simulink model "model_block"  (R2023a)
settings: Solver=VariableStepAuto  StartTime=0.0  StopTime=2  RelTol=1e-3
values from neighbouring files (symbols this model uses):
  C = 660e-6    (= 0.00066)    [execute_model.m]
  duty_cycle = 0.25    [execute_model.m]
  fsw = 15e3    (= 15000)    [execute_model.m]
  L = 200e-6    (= 0.0002)    [execute_model.m]
  R = 10    [execute_model.m]
  vin = 24    [execute_model.m]
libraries: simulink x1
settings Model: Creator=pablo  LastModifiedBy=pablo
settings OptimizationCC: ReuseModelBlockBuffer=off

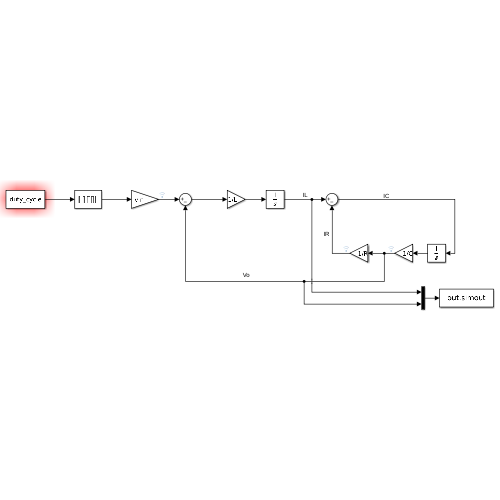
[thumbnail: Simulink's stored preview of the top-level diagram]
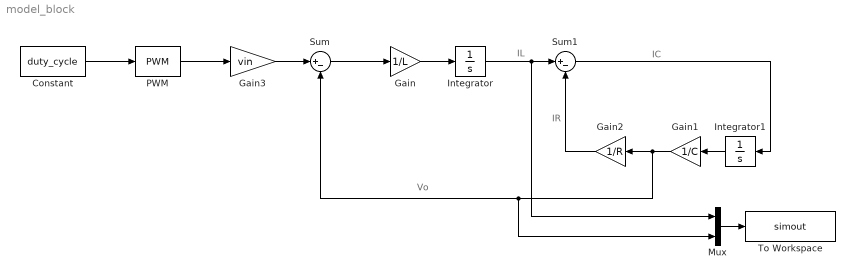
== system model_block ==
  note: IL
  note: IC
  note: IR
  note: Vo
  Constant : Constant  Value=duty_cycle
  Gain : Gain  Gain=1/L
  Gain1 : Gain  Gain=1/C
  Gain2 : Gain  Gain=1/R
  Gain3 : Gain  Gain=vin
  Integrator : Integrator
  Integrator1 : Integrator
  Mux : Mux  Inputs=2
  PWM : simulink/Discontinuities/PWM  DisableCoverage=on  Period=1/fsw  InitialDelay=0  DisallowZeroDutyCycle=off  RunAtFixedTimeIntervals=off  SampleTime=0.1
  Sum : Sum  Inputs=|+-
  Sum1 : Sum  Inputs=|+-
  To Workspace : ToWorkspace  VariableName=simout  SampleTime=-1
      settings: Save2DSignal=2-D array (concatenate along first dimension)
  wires:
  Sum/1 -> Gain/1
  Gain/1 -> Integrator/1
  Integrator/1 -> Mux/1, Sum1/1
  Sum1/1 -> Integrator1/1
  Integrator1/1 -> Gain1/1
  Gain1/1 -> Gain2/1, Mux/2, Sum/2
  Gain2/1 -> Sum1/2
  Gain3/1 -> Sum/1
  PWM/1 -> Gain3/1
  Constant/1 -> PWM/1
  Mux/1 -> To Workspace/1
